simulink model "swim_12B_with_contracts"  (R2019b)
settings: Solver=FixedStepDiscrete  StartTime=0.0  StopTime=10.0  RelTol=1e-3  EnableMultiTasking=on
model workspace (MAT data in the model file):
  ContractValidatorBlocksMap = containers.Map
  ContractValidatorBlocksMap.serialization.keys = {'swim_12B_with_contracts/swim_12B_SWIMSpec/validator'}
  ContractValidatorBlocksMap.serialization.values{1}.block = 'swim_12B_with_contracts/swim_12B_SWIMSpec/validator'
  ContractValidatorBlocksMap.serialization.values{1}.assumePorts = 1
  ContractValidatorBlocksMap.serialization.values{1}.guaranteePorts = 3
  ContractValidatorBlocksMap.serialization.values{1}.modeBlocksPorts = 0
  ContractValidatorBlocksMap.serialization.values{1}.portHandles.Inport = [713.000976562 714.000976562 715.000976562 716.000976562]
  ContractValidatorBlocksMap.serialization.values{1}.portHandles.Outport = 717.000976562
  ContractValidatorBlocksMap.serialization.values{1}.portHandles.Enable = []
  ContractValidatorBlocksMap.serialization.values{1}.portHandles.Trigger = []
  ContractValidatorBlocksMap.serialization.values{1}.portHandles.State = []
  ContractValidatorBlocksMap.serialization.values{1}.portHandles.LConn = []
  ContractValidatorBlocksMap.serialization.values{1}.portHandles.RConn = []
  ContractValidatorBlocksMap.serialization.values{1}.portHandles.Ifaction = []
  ContractValidatorBlocksMap.serialization.values{1}.portHandles.Reset = []
  ContractValidatorBlocksMap.serialization.values{1}.portConnectivity(1).Type = '1'
  ContractValidatorBlocksMap.serialization.values{1}.portConnectivity(1).Position = [1210 730]
  ContractValidatorBlocksMap.serialization.values{1}.portConnectivity(1).SrcBlock = 336.034667969
  ContractValidatorBlocksMap.serialization.values{1}.portConnectivity(1).SrcPort = 0
  ContractValidatorBlocksMap.serialization.values{1}.portConnectivity(1).DstBlock = []
  ContractValidatorBlocksMap.serialization.values{1}.portConnectivity(1).DstPort = []
  ContractValidatorBlocksMap.serialization.values{1}.portConnectivity(2).Type = '2'
  ContractValidatorBlocksMap.serialization.values{1}.portConnectivity(2).Position = [1210 775]
  ContractValidatorBlocksMap.serialization.values{1}.portConnectivity(2).SrcBlock = 340.034667969
  ContractValidatorBlocksMap.serialization.values{1}.portConnectivity(2).SrcPort = 0
  ContractValidatorBlocksMap.serialization.values{1}.portConnectivity(2).DstBlock = []
  ContractValidatorBlocksMap.serialization.values{1}.portConnectivity(2).DstPort = []
  ContractValidatorBlocksMap.serialization.values{1}.portConnectivity(3).Type = '3'
  ContractValidatorBlocksMap.serialization.values{1}.portConnectivity(3).Position = [1210 820]
  ContractValidatorBlocksMap.serialization.values{1}.portConnectivity(3).SrcBlock = 344.034667969
  ContractValidatorBlocksMap.serialization.values{1}.portConnectivity(3).SrcPort = 0
  ContractValidatorBlocksMap.serialization.values{1}.portConnectivity(3).DstBlock = []
  ContractValidatorBlocksMap.serialization.values{1}.portConnectivity(3).DstPort = []
  ContractValidatorBlocksMap.serialization.values{1}.portConnectivity(4).Type = '4'
  ContractValidatorBlocksMap.serialization.values{1}.portConnectivity(4).Position = [1210 865]
  ContractValidatorBlocksMap.serialization.values{1}.portConnectivity(4).SrcBlock = 348.034667969
  ContractValidatorBlocksMap.serialization.values{1}.portConnectivity(4).SrcPort = 0
  ContractValidatorBlocksMap.serialization.values{1}.portConnectivity(4).DstBlock = []
  ContractValidatorBlocksMap.serialization.values{1}.portConnectivity(4).DstPort = []
  ContractValidatorBlocksMap.serialization.values{1}.portConnectivity(5).Type = '1'
  ContractValidatorBlocksMap.serialization.values{1}.portConnectivity(5).Position = [1250 800]
  ContractValidatorBlocksMap.serialization.values{1}.portConnectivity(5).SrcBlock = []
  ContractValidatorBlocksMap.serialization.values{1}.portConnectivity(5).SrcPort = []
  ContractValidatorBlocksMap.serialization.values{1}.portConnectivity(5).DstBlock = 379.034667969
  ContractValidatorBlocksMap.serialization.values{1}.portConnectivity(5).DstPort = 0
  ContractValidatorBlocksMap.serialization.uniformity = 0
  ContractValidatorBlocksMap.serialization.keyType = 'char'
  ContractValidatorBlocksMap.serialization.valueType = 'any'
undefined symbols (not defined in the file): contractAfterSimulation, ContractAssumeBlock, contractBeforeSimulation, ContractBlock, ContractGuaranteeBlock, ContractValidatorBlock, E_DI_CATI, E_DI_DOWN_OR_LOCKED, E_DI_UP_AND_NORMAL, E_MUX_ENABLED, E_OLC_INTERLOCK_NOT_FAILED, E_SWIM_ALLOWED, E_SWIM_NOT_ALLOWED, E_SWIM_WARNING_OFF, E_SWIM_WARNING_ON, saveValidatorParameters
libraries: cocosimLibs x3
settings Model: Creator=belottr  LastModifiedBy=hbourbou
settings DataIOCC: LimitDataPoints=on  SaveFormat=Array  ReturnWorkspaceOutputs=off
settings OptimizationCC: DefaultParameterBehavior=Inlined  ExpressionDepthLimit=2147483647  LifeSpan=inf
settings DebuggingCC: UnderspecifiedInitializationDetection=Classic  MergeDetectMultiDrivingBlocksExec=none  SolverPrmCheckMsg=warning  StateNameClashWarn=warning  SFUnexpectedBacktrackingDiag=warning  SFNoUnconditionalDefaultTransitionDiag=warning  SFExecutionAtInitializationDiag=none  ArithmeticOperatorsInVariantConditions=warning
settings HardwareCC: ProdBitPerPointer=32  ProdBitPerSizeT=32  ProdBitPerPtrDiffT=32  ProdLargestAtomicFloat=None  ProdIntDivRoundTo=Undefined  ProdEndianess=Unspecified  ProdWordSize=32  ProdHWDeviceType=32-bit Generic
settings ModelReferenceCC: UpdateModelReferenceTargets=IfOutOfDate  PropagateSignalLabelsOutOfModel=off
settings SFSimCC: SimUseLocalCustomCode=off  CustomCodeUndefinedFunction=UseInterfaceOnly
settings RTWCC: RTWUseLocalCustomCode=off
settings CodeAppCC: StateflowObjectComments=on
settings GRTTargetCC: TargetLangStandard=C89/C90 (ANSI)  GeneratePreprocessorConditionals=Disable all
settings ConfigComp: CovMetricSettings=dw  CovHtmlReporting=on  CovSaveCumulativeToWorkspaceVar=on  CovSaveSingleToWorkspaceVar=on  CovExternalEMLEnable=off

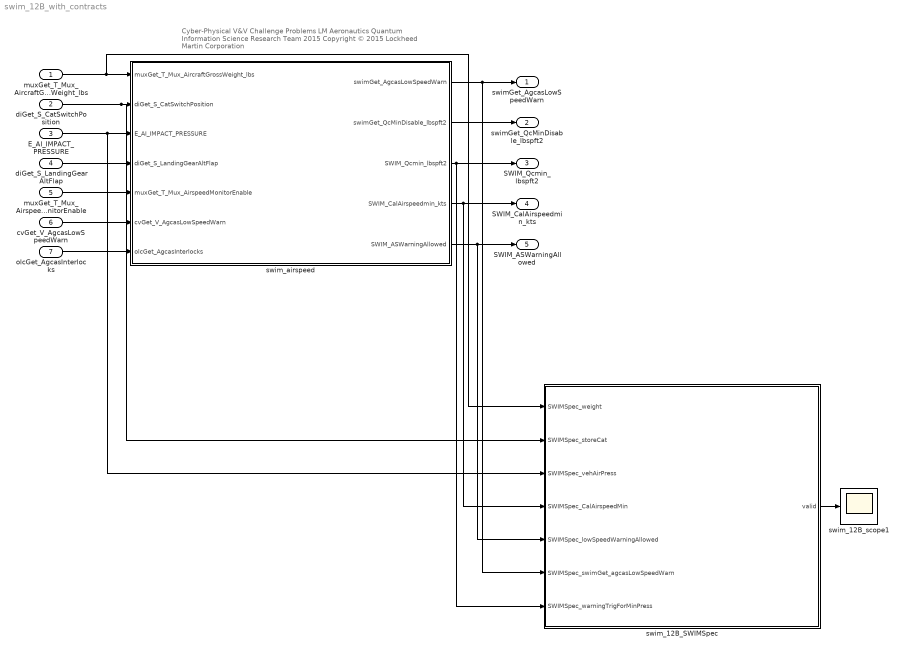
== system swim_12B_with_contracts ==
  note: Cyber-Physical V&V Challenge Problems
      | LM Aeronautics Quantum Information Science Research Team 2015
      | Copyright © 2015 Lockheed Martin Corporation
  muxGet_T_Mux_AircraftGrossWeight_lbs : Inport  OutDataTypeStr=double
  diGet_S_CatSwitchPosition : Inport  Port=2  OutDataTypeStr=int32
  E_AI_IMPACT_PRESSURE : Inport  Port=3  OutDataTypeStr=double
  diGet_S_LandingGearAltFlap : Inport  Port=4  OutDataTypeStr=boolean
  muxGet_T_Mux_AirspeedMonitorEnable : Inport  Port=5  OutDataTypeStr=boolean
  cvGet_V_AgcasLowSpeedWarn : Inport  Port=6  OutDataTypeStr=boolean
  olcGet_AgcasInterlocks : Inport  Port=7  OutDataTypeStr=boolean
  swim_12B_SWIMSpec : Subsystem  mask(ContractBlock){ContractBlockType=ContractBlock}
      mask init:
      | set_param(gcb, 'LinkStatus', 'none');
      mask DialogControl DescTextVar Prompt: Contract block
      mask Display:
      | text(0.5, 0.5, '{\bf\fontsize{20}Contract}', 'hor', 'center', 'texmode','on');
      | blocks = find_system(gcb, 'LookUnderMasks','all', 'SearchDepth',1,'BlockType','Inport');
      | for i = 1 : length(blocks)
      |     blockName = get_param(blocks(i), 'Name');
      |     [path, blockName] = fileparts(char(blockName));
      |     port_label('input', i, blockName);
      | end
      | 
      | blocks = find_system(gcb, 'LookUnderMasks','all', 'SearchDepth',1,'BlockType','Outport');
      | for i = 1 : length(blocks)
      |     blockName = get_param(blocks(i), 'Name');
      |     [path, blockName] = fileparts(char(blockName));
      |     port_label('output', i, blockName);
      | end
  swim_12B_scope1 : Scope
  swim_airspeed : Subsystem
  swimGet_AgcasLowSpeedWarn : Outport  VectorParamsAs1DForOutWhenUnconnected=off
  swimGet_QcMinDisable_lbspft2 : Outport  Port=2  VectorParamsAs1DForOutWhenUnconnected=off
  SWIM_Qcmin_lbspft2 : Outport  Port=3  VectorParamsAs1DForOutWhenUnconnected=off
  SWIM_CalAirspeedmin_kts : Outport  Port=4  VectorParamsAs1DForOutWhenUnconnected=off
  SWIM_ASWarningAllowed : Outport  Port=5  VectorParamsAs1DForOutWhenUnconnected=off
  wires:
  muxGet_T_Mux_AircraftGrossWeight_lbs/1 -> swim_airspeed/1(muxGet_T_Mux_AircraftGrossWeight_lbs), swim_12B_SWIMSpec/1(SWIMSpec_weight)
  diGet_S_CatSwitchPosition/1 -> swim_airspeed/2(diGet_S_CatSwitchPosition), swim_12B_SWIMSpec/2(SWIMSpec_storeCat)
  E_AI_IMPACT_PRESSURE/1 -> swim_airspeed/3(E_AI_IMPACT_PRESSURE), swim_12B_SWIMSpec/3(SWIMSpec_vehAirPress)
  diGet_S_LandingGearAltFlap/1 -> swim_airspeed/4(diGet_S_LandingGearAltFlap)
  muxGet_T_Mux_AirspeedMonitorEnable/1 -> swim_airspeed/5(muxGet_T_Mux_AirspeedMonitorEnable)
  cvGet_V_AgcasLowSpeedWarn/1 -> swim_airspeed/6(cvGet_V_AgcasLowSpeedWarn)
  olcGet_AgcasInterlocks/1 -> swim_airspeed/7(olcGet_AgcasInterlocks)
  swim_airspeed/3(SWIM_Qcmin_lbspft2) -> SWIM_Qcmin_lbspft2/1, swim_12B_SWIMSpec/7(SWIMSpec_warningTrigForMinPress)
  swim_airspeed/2(swimGet_QcMinDisable_lbspft2) -> swimGet_QcMinDisable_lbspft2/1
  swim_airspeed/1(swimGet_AgcasLowSpeedWarn) -> swim_12B_SWIMSpec/6(SWIMSpec_swimGet_agcasLowSpeedWarn), swimGet_AgcasLowSpeedWarn/1
  swim_airspeed/4(SWIM_CalAirspeedmin_kts) -> SWIM_CalAirspeedmin_kts/1, swim_12B_SWIMSpec/4(SWIMSpec_CalAirspeedMin)
  swim_airspeed/5(SWIM_ASWarningAllowed) -> SWIM_ASWarningAllowed/1, swim_12B_SWIMSpec/5(SWIMSpec_lowSpeedWarningAllowed)
  swim_12B_SWIMSpec/1(valid) -> swim_12B_scope1/1

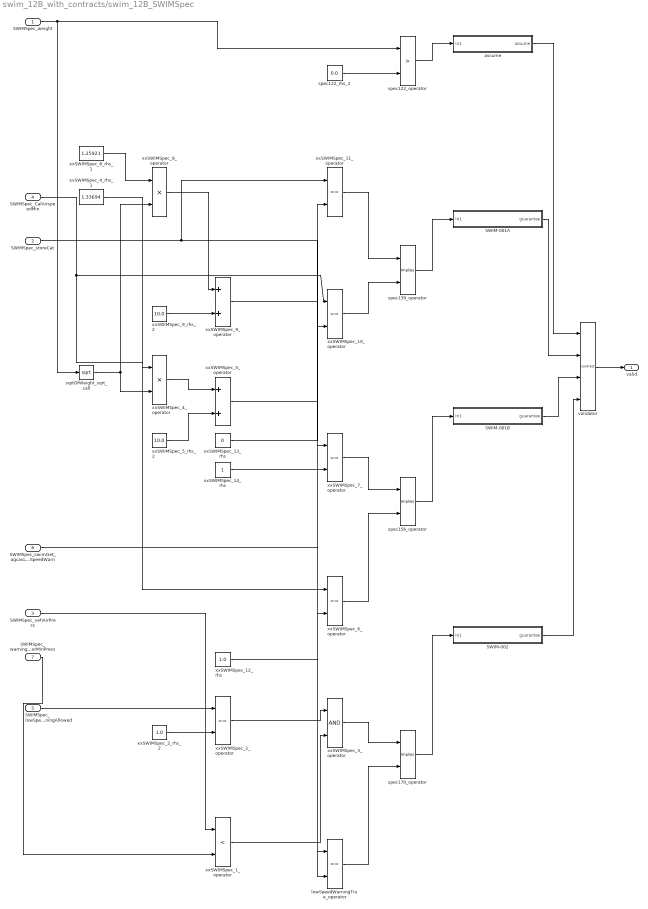
== system swim_12B_with_contracts/swim_12B_SWIMSpec ==
  SWIMSpec_weight : Inport  OutDataTypeStr=double
  SWIMSpec_storeCat : Inport  Port=2
  SWIMSpec_vehAirPress : Inport  Port=3  OutDataTypeStr=double
  SWIMSpec_CalAirspeedMin : Inport  Port=4  OutDataTypeStr=double
  SWIMSpec_lowSpeedWarningAllowed : Inport  Port=5  OutDataTypeStr=double
  SWIMSpec_swimGet_agcasLowSpeedWarn : Inport  Port=6  OutDataTypeStr=double
  SWIMSpec_warningTrigForMinPress : Inport  Port=7  OutDataTypeStr=double
  SWIM-001A : Subsystem  mask(ContractGuaranteeBlock){ContractBlockType=ContractGuaranteeBlock}
      mask init:
      | set_param(gcb, 'LinkStatus', 'none');
      mask DialogControl DescTextVar Prompt: Guarantee block
  SWIM-001B : Subsystem  mask(ContractGuaranteeBlock){ContractBlockType=ContractGuaranteeBlock}
      mask init:
      | set_param(gcb, 'LinkStatus', 'none');
      mask DialogControl DescTextVar Prompt: Guarantee block
  SWIM-002 : Subsystem  mask(ContractGuaranteeBlock){ContractBlockType=ContractGuaranteeBlock}
      mask init:
      | set_param(gcb, 'LinkStatus', 'none');
      mask DialogControl DescTextVar Prompt: Guarantee block
  assume : Subsystem  mask(ContractAssumeBlock){ContractBlockType=ContractAssumeBlock}
      mask init:
      | set_param(gcb, 'LinkStatus', 'none');
      mask DialogControl DescTextVar Prompt: Assume block
  lowSpeedWarningTrue_operator : RelationalOperator  Operator===  OutDataTypeStr=boolean  RndMeth=Simplest
  spec122_operator : RelationalOperator  Operator=>  OutDataTypeStr=boolean  RndMeth=Simplest
  spec122_rhs_2 : Constant  Value=0.0  OutDataTypeStr=double
  spec139_operator : cocosimLibs/Implies  SystemSampleTime=-1  Latency=0  AutoFrameSizeCalculation=off
  spec156_operator : cocosimLibs/Implies  SystemSampleTime=-1  Latency=0  AutoFrameSizeCalculation=off
  spec170_operator : cocosimLibs/Implies  SystemSampleTime=-1  Latency=0  AutoFrameSizeCalculation=off
  sqrtOfWeight_sqrt_call : Sqrt  SaturateOnIntegerOverflow=on
  validator : M-S-Function  LoadFcn=saveValidatorParameters(gcb);  InitFcn=contractBeforeSimulation();  StopFcn=contractAfterSimulation();  FunctionName=contract  mask(ContractValidatorBlock){assumePorts=1, guaranteePorts=3, modePorts=0, ContractBlockType=ContractValidatorBlock, createInportsCheckbox=off}
      mask prompts: assumePorts "Assume ports     :"; guaranteePorts "Guarantee ports :"; modePorts "Mode ports        :"; createInportsCheckbox "Create inports and connect them automatically"
      mask init:
      | set_param(gcb,'LinkStatus','none');
      | contract_callback('inputs_callback',gcb);
      mask DialogControl DescTextVar Prompt: The validator block implements the following logic: <br> <br> <b>Sofar</b>(assume<sub>1</sub> <b>&#8743;</b> assume<sub>2</sub> <b>&#8743;</b> ... assume<sub>k</sub>) <b>&rarr;</b> (guarantee<sub>1</sub> <b>&#8743;</b> guarantee<sub>2</sub> <b>&#8743;</b> ... guarantee<sub>m</sub> <b>&#8743;</b>  mode<sub>1</sub> <b>&#8743;</b> mode<sub>2</sub> <b>&#8743;</b> ... <b>&#8743;</b> mode<sub>n</sub> )<br> where mode<sub>i</sub> = require<sub>i</sub> <b>&rarr;</b> ensure<sub>i</sub>
      mask Display:
      | color('black');
      | port_label('input',1,'assume');
      | port_label('input',2,'guarantee');
      | port_label('input',3,'guarantee');
      | port_label('input',4,'guarantee');
      | port_label('output',1,'valid');
  xxSWIMSpec_10_operator : RelationalOperator  Operator===  OutDataTypeStr=boolean  RndMeth=Simplest
  xxSWIMSpec_11_operator : RelationalOperator  Operator===  OutDataTypeStr=boolean  RndMeth=Simplest
  xxSWIMSpec_12_rhs : Constant  Value=1.0  OutDataTypeStr=double
  xxSWIMSpec_13_rhs : Constant  Value=0  OutDataTypeStr=Inherit: Inherit via back propagation
  xxSWIMSpec_14_rhs : Constant  OutDataTypeStr=Inherit: Inherit via back propagation
  xxSWIMSpec_1_operator : RelationalOperator  Operator=<  OutDataTypeStr=boolean  RndMeth=Simplest
  xxSWIMSpec_2_operator : RelationalOperator  Operator===  OutDataTypeStr=boolean  RndMeth=Simplest
  xxSWIMSpec_2_rhs_2 : Constant  Value=1.0  OutDataTypeStr=double
  xxSWIMSpec_3_operator : Logic  AllPortsSameDT=off  OutDataTypeStr=boolean
  xxSWIMSpec_4_operator : Product  OutDataTypeStr=double
  xxSWIMSpec_4_rhs_1 : Constant  Value=1.33694  OutDataTypeStr=double
  xxSWIMSpec_5_operator : Sum  OutDataTypeStr=double
  xxSWIMSpec_5_rhs_2 : Constant  Value=10.0  OutDataTypeStr=double
  xxSWIMSpec_6_operator : RelationalOperator  Operator===  OutDataTypeStr=boolean  RndMeth=Simplest
  xxSWIMSpec_7_operator : RelationalOperator  Operator===  OutDataTypeStr=boolean  RndMeth=Simplest
  xxSWIMSpec_8_operator : Product  OutDataTypeStr=double
  xxSWIMSpec_8_rhs_1 : Constant  Value=1.25921  OutDataTypeStr=double
  xxSWIMSpec_9_operator : Sum  OutDataTypeStr=double
  xxSWIMSpec_9_rhs_2 : Constant  Value=10.0  OutDataTypeStr=double
  valid : Outport
  wires:
  validator/1 -> valid/1
  xxSWIMSpec_9_rhs_2/1 -> xxSWIMSpec_9_operator/2
  xxSWIMSpec_8_operator/1 -> xxSWIMSpec_9_operator/1
  xxSWIMSpec_8_rhs_1/1 -> xxSWIMSpec_8_operator/1
  xxSWIMSpec_14_rhs/1 -> xxSWIMSpec_7_operator/2
  xxSWIMSpec_5_operator/1 -> xxSWIMSpec_6_operator/2
  xxSWIMSpec_5_rhs_2/1 -> xxSWIMSpec_5_operator/2
  xxSWIMSpec_4_operator/1 -> xxSWIMSpec_5_operator/1
  xxSWIMSpec_4_rhs_1/1 -> xxSWIMSpec_4_operator/1
  xxSWIMSpec_1_operator/1 -> xxSWIMSpec_3_operator/2
  xxSWIMSpec_2_operator/1 -> xxSWIMSpec_3_operator/1
  xxSWIMSpec_2_rhs_2/1 -> xxSWIMSpec_2_operator/2
  SWIMSpec_lowSpeedWarningAllowed/1 -> xxSWIMSpec_2_operator/1
  SWIMSpec_warningTrigForMinPress/1 -> xxSWIMSpec_1_operator/2
  SWIMSpec_vehAirPress/1 -> xxSWIMSpec_1_operator/1
  xxSWIMSpec_13_rhs/1 -> xxSWIMSpec_11_operator/2
  xxSWIMSpec_9_operator/1 -> xxSWIMSpec_10_operator/2
  SWIM-002/1(guarantee) -> validator/4
  SWIM-001B/1(guarantee) -> validator/3
  SWIM-001A/1(guarantee) -> validator/2
  assume/1(assume) -> validator/1
  lowSpeedWarningTrue_operator/1 -> spec170_operator/2
  xxSWIMSpec_3_operator/1 -> spec170_operator/1
  xxSWIMSpec_6_operator/1 -> spec156_operator/2
  xxSWIMSpec_7_operator/1 -> spec156_operator/1
  xxSWIMSpec_10_operator/1 -> spec139_operator/2
  xxSWIMSpec_11_operator/1 -> spec139_operator/1
  spec122_rhs_2/1 -> spec122_operator/2
  xxSWIMSpec_12_rhs/1 -> lowSpeedWarningTrue_operator/2
  SWIMSpec_swimGet_agcasLowSpeedWarn/1 -> lowSpeedWarningTrue_operator/1
  spec170_operator/1 -> SWIM-002/1(In1)
  spec156_operator/1 -> SWIM-001B/1(In1)
  spec139_operator/1 -> SWIM-001A/1(In1)
  spec122_operator/1 -> assume/1(In1)
  SWIMSpec_weight/1 -> sqrtOfWeight_sqrt_call/1, spec122_operator/1
  SWIMSpec_CalAirspeedMin/1 -> xxSWIMSpec_6_operator/1, xxSWIMSpec_10_operator/1
  SWIMSpec_storeCat/1 -> xxSWIMSpec_7_operator/1, xxSWIMSpec_11_operator/1
  sqrtOfWeight_sqrt_call/1 -> xxSWIMSpec_8_operator/2, xxSWIMSpec_4_operator/2

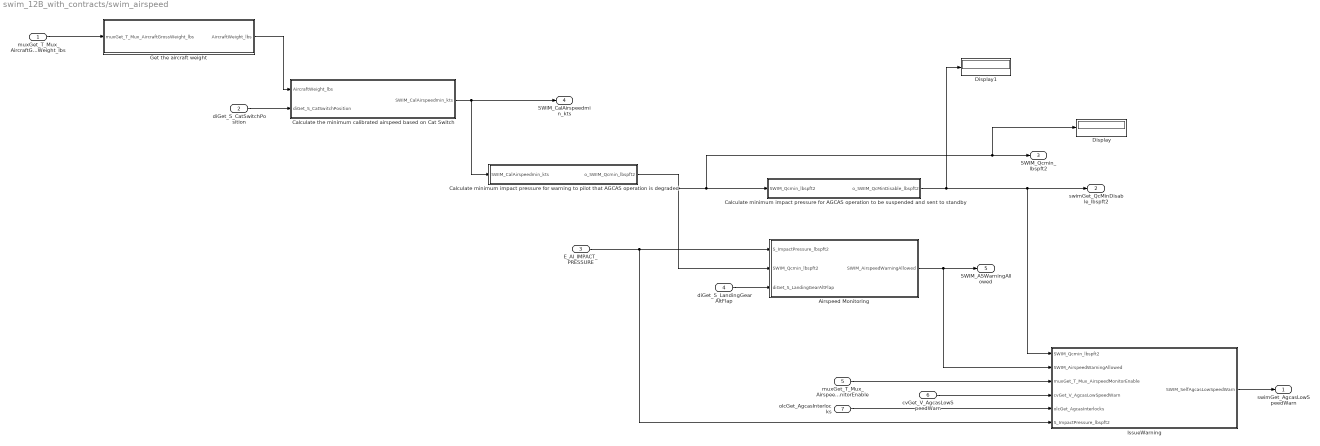
== system swim_12B_with_contracts/swim_airspeed ==
  muxGet_T_Mux_AircraftGrossWeight_lbs : Inport
  diGet_S_CatSwitchPosition : Inport  Port=2
  E_AI_IMPACT_PRESSURE : Inport  Port=3
  diGet_S_LandingGearAltFlap : Inport  Port=4
  muxGet_T_Mux_AirspeedMonitorEnable : Inport  Port=5
  cvGet_V_AgcasLowSpeedWarn : Inport  Port=6
  olcGet_AgcasInterlocks : Inport  Port=7
  Airspeed Monitoring : Subsystem
  Calculate minimum impact pressure for AGCAS operation to be suspended and sent to standby : Subsystem
  Calculate minimum impact pressure for warning to pilot that AGCAS operation is degraded : Subsystem
  Calculate the minimum calibrated airspeed based on Cat Switch : Subsystem
  Display : Display
  Display1 : Display
  Get the aircraft weight : Subsystem
  IssueWarning : Subsystem
  swimGet_AgcasLowSpeedWarn : Outport  VectorParamsAs1DForOutWhenUnconnected=off
  swimGet_QcMinDisable_lbspft2 : Outport  Port=2  VectorParamsAs1DForOutWhenUnconnected=off
  SWIM_Qcmin_lbspft2 : Outport  Port=3  VectorParamsAs1DForOutWhenUnconnected=off
  SWIM_CalAirspeedmin_kts : Outport  Port=4  VectorParamsAs1DForOutWhenUnconnected=off
  SWIM_ASWarningAllowed : Outport  Port=5  VectorParamsAs1DForOutWhenUnconnected=off
  wires:
  muxGet_T_Mux_AircraftGrossWeight_lbs/1 -> Get the aircraft weight/1(muxGet_T_Mux_AircraftGrossWeight_lbs)
  diGet_S_CatSwitchPosition/1 -> Calculate the minimum calibrated airspeed based on Cat Switch/2(diGet_S_CatSwitchPosition)
  Get the aircraft weight/1(AircraftWeight_lbs) -> Calculate the minimum calibrated airspeed based on Cat Switch/1(AircraftWeight_lbs)
  Calculate the minimum calibrated airspeed based on Cat Switch/1(SWIM_CalAirspeedmin_kts) -> Calculate minimum impact pressure for warning to pilot that AGCAS operation is degraded/1(SWIM_CalAirspeedmin_kts), SWIM_CalAirspeedmin_kts/1
  E_AI_IMPACT_PRESSURE/1 -> IssueWarning/6(S_ImpactPressure_lbspft2), Airspeed Monitoring/1(S_ImpactPressure_lbspft2)
  diGet_S_LandingGearAltFlap/1 -> Airspeed Monitoring/3(diGet_S_LandingGearAltFlap)
  IssueWarning/1(SWIM_SelfAgcasLowSpeedWarn) -> swimGet_AgcasLowSpeedWarn/1
  muxGet_T_Mux_AirspeedMonitorEnable/1 -> IssueWarning/3(muxGet_T_Mux_AirspeedMonitorEnable)
  cvGet_V_AgcasLowSpeedWarn/1 -> IssueWarning/4(cvGet_V_AgcasLowSpeedWarn)
  olcGet_AgcasInterlocks/1 -> IssueWarning/5(olcGet_AgcasInterlocks)
  Calculate minimum impact pressure for AGCAS operation to be suspended and sent to standby/1(o_SWIM_QcMinDisable_lbspft2) -> Display1/1, IssueWarning/1(SWIM_Qcmin_lbspft2), swimGet_QcMinDisable_lbspft2/1
  Airspeed Monitoring/1(SWIM_AirspeedWarningAllowed) -> IssueWarning/2(SWIM_AirspeedWarningAllowed), SWIM_ASWarningAllowed/1
  Calculate minimum impact pressure for warning to pilot that AGCAS operation is degraded/1(o_SWIM_Qcmin_lbspft2) -> Airspeed Monitoring/2(SWIM_Qcmin_lbspft2), Display/1, SWIM_Qcmin_lbspft2/1, Calculate minimum impact pressure for AGCAS operation to be suspended and sent to standby/1(SWIM_Qcmin_lbspft2)

== system swim_12B_with_contracts/swim_12B_SWIMSpec/SWIM-001A ==
  In1 : Inport
  guarantee : Outport  OutDataTypeStr=boolean
  wires:
  In1/1 -> guarantee/1

== system swim_12B_with_contracts/swim_12B_SWIMSpec/SWIM-001B ==
  In1 : Inport
  guarantee : Outport  OutDataTypeStr=boolean
  wires:
  In1/1 -> guarantee/1

== system swim_12B_with_contracts/swim_12B_SWIMSpec/SWIM-002 ==
  In1 : Inport
  guarantee : Outport  OutDataTypeStr=boolean
  wires:
  In1/1 -> guarantee/1

== system swim_12B_with_contracts/swim_12B_SWIMSpec/assume ==
  In1 : Inport
  assume : Outport  OutDataTypeStr=boolean
  wires:
  In1/1 -> assume/1

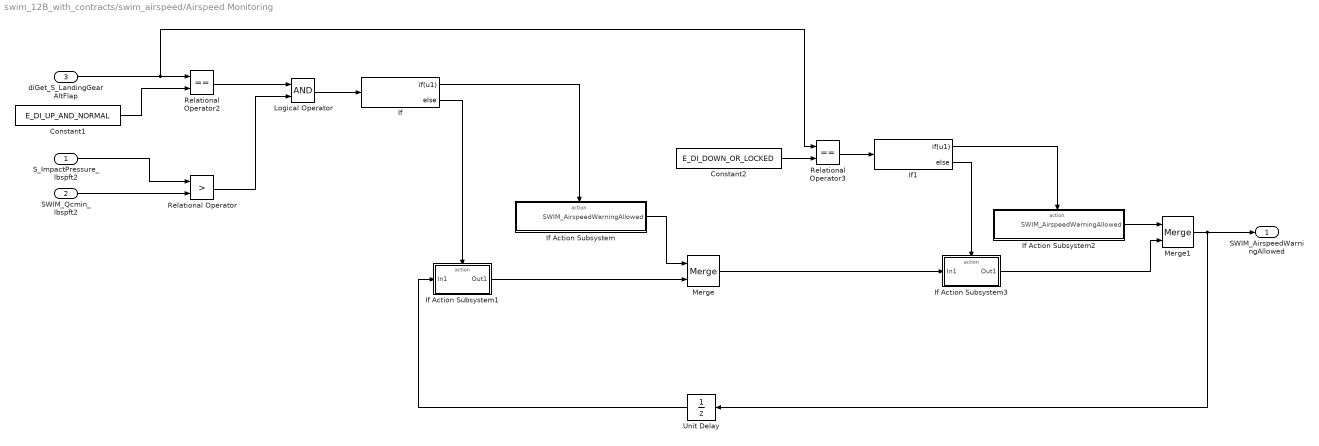
== system swim_12B_with_contracts/swim_airspeed/Airspeed Monitoring ==
  S_ImpactPressure_lbspft2 : Inport
  SWIM_Qcmin_lbspft2 : Inport  Port=2
  diGet_S_LandingGearAltFlap : Inport  Port=3
  Constant1 : Constant  Value=E_DI_UP_AND_NORMAL
  Constant2 : Constant  Value=E_DI_DOWN_OR_LOCKED
  If : If  IfExpression=u1
  If Action Subsystem : Subsystem  TreatAsAtomicUnit=on
  If Action Subsystem1 : Subsystem  TreatAsAtomicUnit=on
  If Action Subsystem2 : Subsystem  TreatAsAtomicUnit=on
  If Action Subsystem3 : Subsystem  TreatAsAtomicUnit=on
  If1 : If  IfExpression=u1
  Logical Operator : Logic  AllPortsSameDT=off  OutDataTypeStr=boolean
  Merge : Merge
  Merge1 : Merge
  Relational Operator : RelationalOperator  Operator=>  OutDataTypeStr=boolean  RndMeth=Nearest
  Relational Operator2 : RelationalOperator  Operator===  OutDataTypeStr=boolean  RndMeth=Nearest
  Relational Operator3 : RelationalOperator  Operator===  OutDataTypeStr=boolean  RndMeth=Nearest
  Unit Delay : UnitDelay  InitialCondition=E_SWIM_NOT_ALLOWED  SampleTime=-1  HasFrameUpgradeWarning=on
  SWIM_AirspeedWarningAllowed : Outport  VectorParamsAs1DForOutWhenUnconnected=off
  wires:
  S_ImpactPressure_lbspft2/1 -> Relational Operator/1
  SWIM_Qcmin_lbspft2/1 -> Relational Operator/2
  diGet_S_LandingGearAltFlap/1 -> Relational Operator3/1, Relational Operator2/1
  Constant1/1 -> Relational Operator2/2
  If/1 -> If Action Subsystem/Action
  If/2 -> If Action Subsystem1/Action
  If Action Subsystem/1(SWIM_AirspeedWarningAllowed) -> Merge/1
  If Action Subsystem1/1(Out1) -> Merge/2
  Constant2/1 -> Relational Operator3/2
  Relational Operator3/1 -> If1/1
  Relational Operator/1 -> Logical Operator/2
  Relational Operator2/1 -> Logical Operator/1
  Logical Operator/1 -> If/1
  If1/1 -> If Action Subsystem2/Action
  If1/2 -> If Action Subsystem3/Action
  If Action Subsystem2/1(SWIM_AirspeedWarningAllowed) -> Merge1/1
  If Action Subsystem3/1(Out1) -> Merge1/2
  Merge/1 -> If Action Subsystem3/1(In1)
  Merge1/1 -> Unit Delay/1, SWIM_AirspeedWarningAllowed/1
  Unit Delay/1 -> If Action Subsystem1/1(In1)

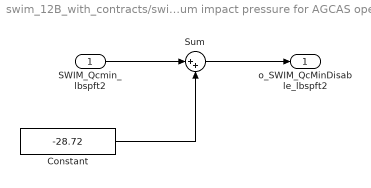
== system swim_12B_with_contracts/swim_airspeed/Calculate minimum impact pressure for AGCAS operation to be suspended and sent to standby ==
  SWIM_Qcmin_lbspft2 : Inport
  Constant : Constant  Value=-28.72
  Sum : Sum  Inputs=|++
  o_SWIM_QcMinDisable_lbspft2 : Outport  VectorParamsAs1DForOutWhenUnconnected=off
  wires:
  SWIM_Qcmin_lbspft2/1 -> Sum/1
  Constant/1 -> Sum/2
  Sum/1 -> o_SWIM_QcMinDisable_lbspft2/1

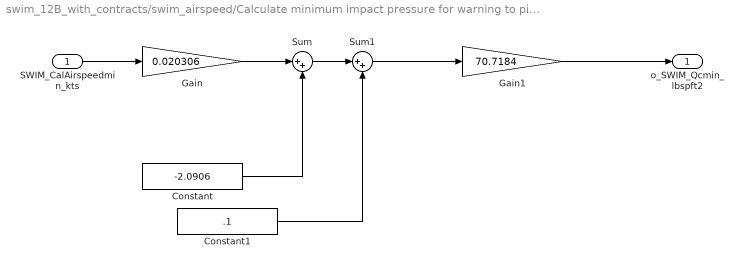
== system swim_12B_with_contracts/swim_airspeed/Calculate minimum impact pressure for warning to pilot that AGCAS operation is degraded ==
  SWIM_CalAirspeedmin_kts : Inport
  Constant : Constant  Value=-2.0906
  Constant1 : Constant  Value=.1
  Gain : Gain  Gain=0.020306
  Gain1 : Gain  Gain=70.7184
  Sum : Sum  Inputs=|++
  Sum1 : Sum  Inputs=|++
  o_SWIM_Qcmin_lbspft2 : Outport  VectorParamsAs1DForOutWhenUnconnected=off
  wires:
  SWIM_CalAirspeedmin_kts/1 -> Gain/1
  Gain/1 -> Sum/1
  Constant/1 -> Sum/2
  Sum/1 -> Sum1/1
  Constant1/1 -> Sum1/2
  Sum1/1 -> Gain1/1
  Gain1/1 -> o_SWIM_Qcmin_lbspft2/1

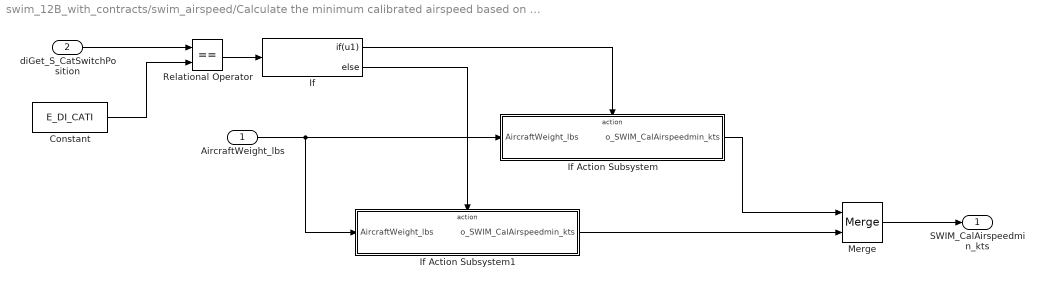
== system swim_12B_with_contracts/swim_airspeed/Calculate the minimum calibrated airspeed based on Cat Switch ==
  AircraftWeight_lbs : Inport
  diGet_S_CatSwitchPosition : Inport  Port=2
  Constant : Constant  Value=E_DI_CATI
  If : If  IfExpression=u1
  If Action Subsystem : Subsystem  TreatAsAtomicUnit=on
  If Action Subsystem1 : Subsystem  TreatAsAtomicUnit=on
  Merge : Merge
  Relational Operator : RelationalOperator  Operator===  OutDataTypeStr=boolean  RndMeth=Nearest
  SWIM_CalAirspeedmin_kts : Outport  VectorParamsAs1DForOutWhenUnconnected=off
  wires:
  If/1 -> If Action Subsystem/Action
  If/2 -> If Action Subsystem1/Action
  If Action Subsystem/1(o_SWIM_CalAirspeedmin_kts) -> Merge/1
  If Action Subsystem1/1(o_SWIM_CalAirspeedmin_kts) -> Merge/2
  Merge/1 -> SWIM_CalAirspeedmin_kts/1
  AircraftWeight_lbs/1 -> If Action Subsystem/1(AircraftWeight_lbs), If Action Subsystem1/1(AircraftWeight_lbs)
  Constant/1 -> Relational Operator/2
  diGet_S_CatSwitchPosition/1 -> Relational Operator/1
  Relational Operator/1 -> If/1

== system swim_12B_with_contracts/swim_airspeed/Get the aircraft weight ==
  muxGet_T_Mux_AircraftGrossWeight_lbs : Inport
  AircraftWeight_lbs : Outport  VectorParamsAs1DForOutWhenUnconnected=off
  wires:
  muxGet_T_Mux_AircraftGrossWeight_lbs/1 -> AircraftWeight_lbs/1

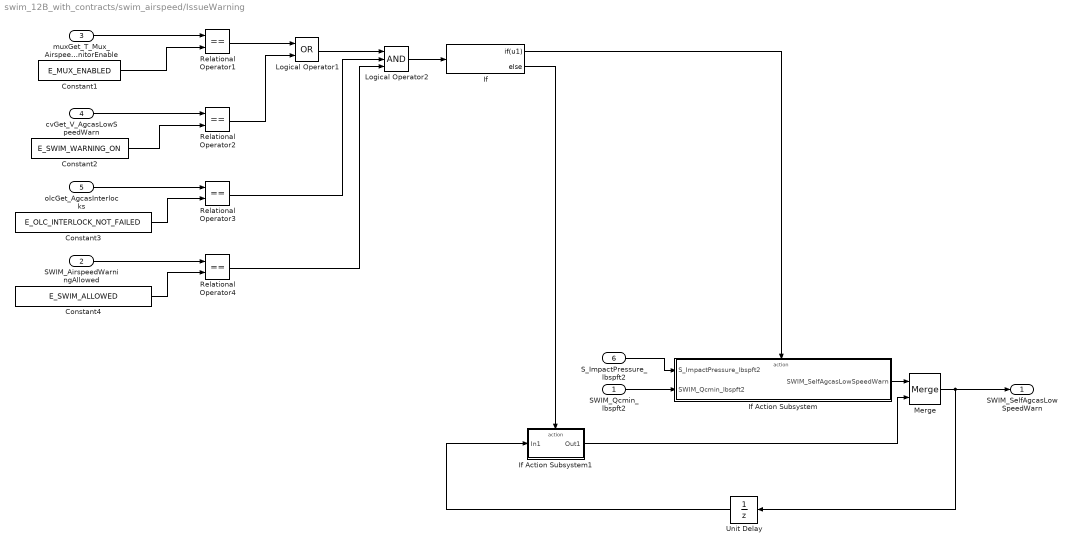
== system swim_12B_with_contracts/swim_airspeed/IssueWarning ==
  SWIM_Qcmin_lbspft2 : Inport
  SWIM_AirspeedWarningAllowed : Inport  Port=2
  muxGet_T_Mux_AirspeedMonitorEnable : Inport  Port=3
  cvGet_V_AgcasLowSpeedWarn : Inport  Port=4
  olcGet_AgcasInterlocks : Inport  Port=5
  S_ImpactPressure_lbspft2 : Inport  Port=6
  Constant1 : Constant  Value=E_MUX_ENABLED
  Constant2 : Constant  Value=E_SWIM_WARNING_ON
  Constant3 : Constant  Value=E_OLC_INTERLOCK_NOT_FAILED
  Constant4 : Constant  Value=E_SWIM_ALLOWED
  If : If  IfExpression=u1
  If Action Subsystem : Subsystem  TreatAsAtomicUnit=on
  If Action Subsystem1 : Subsystem  TreatAsAtomicUnit=on
  Logical Operator1 : Logic  Operator=OR  AllPortsSameDT=off  OutDataTypeStr=boolean
  Logical Operator2 : Logic  Inputs=3  AllPortsSameDT=off  OutDataTypeStr=boolean
  Merge : Merge
  Relational Operator{1..4} (4 alike) : RelationalOperator  Operator===  OutDataTypeStr=boolean  RndMeth=Nearest
  Unit Delay : UnitDelay  InitialCondition=E_SWIM_WARNING_OFF  SampleTime=-1  HasFrameUpgradeWarning=on
  SWIM_SelfAgcasLowSpeedWarn : Outport  VectorParamsAs1DForOutWhenUnconnected=off
  wires:
  muxGet_T_Mux_AirspeedMonitorEnable/1 -> Relational Operator1/1
  cvGet_V_AgcasLowSpeedWarn/1 -> Relational Operator2/1
  Constant2/1 -> Relational Operator2/2
  Constant1/1 -> Relational Operator1/2
  olcGet_AgcasInterlocks/1 -> Relational Operator3/1
  Constant3/1 -> Relational Operator3/2
  SWIM_AirspeedWarningAllowed/1 -> Relational Operator4/1
  Constant4/1 -> Relational Operator4/2
  Relational Operator1/1 -> Logical Operator1/1
  Relational Operator2/1 -> Logical Operator1/2
  Logical Operator1/1 -> Logical Operator2/1
  Relational Operator3/1 -> Logical Operator2/2
  Relational Operator4/1 -> Logical Operator2/3
  Logical Operator2/1 -> If/1
  If/1 -> If Action Subsystem/Action
  If/2 -> If Action Subsystem1/Action
  SWIM_Qcmin_lbspft2/1 -> If Action Subsystem/2(SWIM_Qcmin_lbspft2)
  If Action Subsystem/1(SWIM_SelfAgcasLowSpeedWarn) -> Merge/1
  Merge/1 -> Unit Delay/1, SWIM_SelfAgcasLowSpeedWarn/1
  If Action Subsystem1/1(Out1) -> Merge/2
  Unit Delay/1 -> If Action Subsystem1/1(In1)
  S_ImpactPressure_lbspft2/1 -> If Action Subsystem/1(S_ImpactPressure_lbspft2)

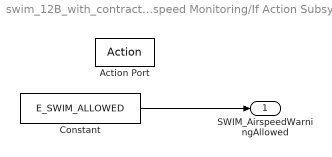
== system swim_12B_with_contracts/swim_airspeed/Airspeed Monitoring/If Action Subsystem ==
  Action Port : ActionPort  ActionPortLabel=if(u1)
  Constant : Constant  Value=E_SWIM_ALLOWED
  SWIM_AirspeedWarningAllowed : Outport  VectorParamsAs1DForOutWhenUnconnected=off
  wires:
  Constant/1 -> SWIM_AirspeedWarningAllowed/1

== system swim_12B_with_contracts/swim_airspeed/Airspeed Monitoring/If Action Subsystem1 ==
  In1 : Inport
  Action Port : ActionPort  ActionPortLabel=else
  Out1 : Outport  VectorParamsAs1DForOutWhenUnconnected=off
  wires:
  In1/1 -> Out1/1

== system swim_12B_with_contracts/swim_airspeed/Airspeed Monitoring/If Action Subsystem2 ==
  Action Port : ActionPort  ActionPortLabel=if(u1)
  Constant : Constant  Value=E_SWIM_NOT_ALLOWED
  SWIM_AirspeedWarningAllowed : Outport  VectorParamsAs1DForOutWhenUnconnected=off
  wires:
  Constant/1 -> SWIM_AirspeedWarningAllowed/1

== system swim_12B_with_contracts/swim_airspeed/Airspeed Monitoring/If Action Subsystem3 ==
  In1 : Inport
  Action Port : ActionPort  ActionPortLabel=else
  Out1 : Outport  VectorParamsAs1DForOutWhenUnconnected=off
  wires:
  In1/1 -> Out1/1

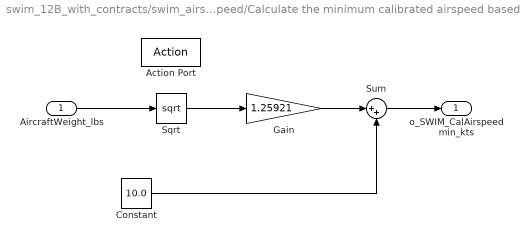
== system swim_12B_with_contracts/swim_airspeed/Calculate the minimum calibrated airspeed based on Cat Switch/If Action Subsystem ==
  AircraftWeight_lbs : Inport
  Action Port : ActionPort  ActionPortLabel=if(u1)
  Constant : Constant  Value=10.0
  Gain : Gain  Gain=1.25921
  Sqrt : Sqrt  SaturateOnIntegerOverflow=on
  Sum : Sum  Inputs=|++
  o_SWIM_CalAirspeedmin_kts : Outport  VectorParamsAs1DForOutWhenUnconnected=off
  wires:
  AircraftWeight_lbs/1 -> Sqrt/1
  Gain/1 -> Sum/1
  Constant/1 -> Sum/2
  Sum/1 -> o_SWIM_CalAirspeedmin_kts/1
  Sqrt/1 -> Gain/1

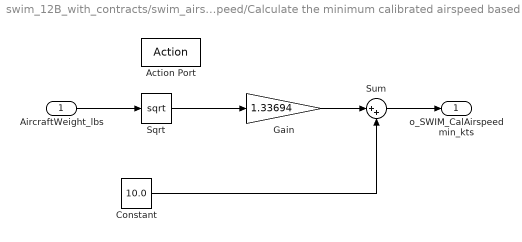
== system swim_12B_with_contracts/swim_airspeed/Calculate the minimum calibrated airspeed based on Cat Switch/If Action Subsystem1 ==
  AircraftWeight_lbs : Inport
  Action Port : ActionPort  ActionPortLabel=else
  Constant : Constant  Value=10.0
  Gain : Gain  Gain=1.33694
  Sqrt : Sqrt  SaturateOnIntegerOverflow=on
  Sum : Sum  Inputs=|++
  o_SWIM_CalAirspeedmin_kts : Outport  VectorParamsAs1DForOutWhenUnconnected=off
  wires:
  Sum/1 -> o_SWIM_CalAirspeedmin_kts/1
  Constant/1 -> Sum/2
  Gain/1 -> Sum/1
  AircraftWeight_lbs/1 -> Sqrt/1
  Sqrt/1 -> Gain/1

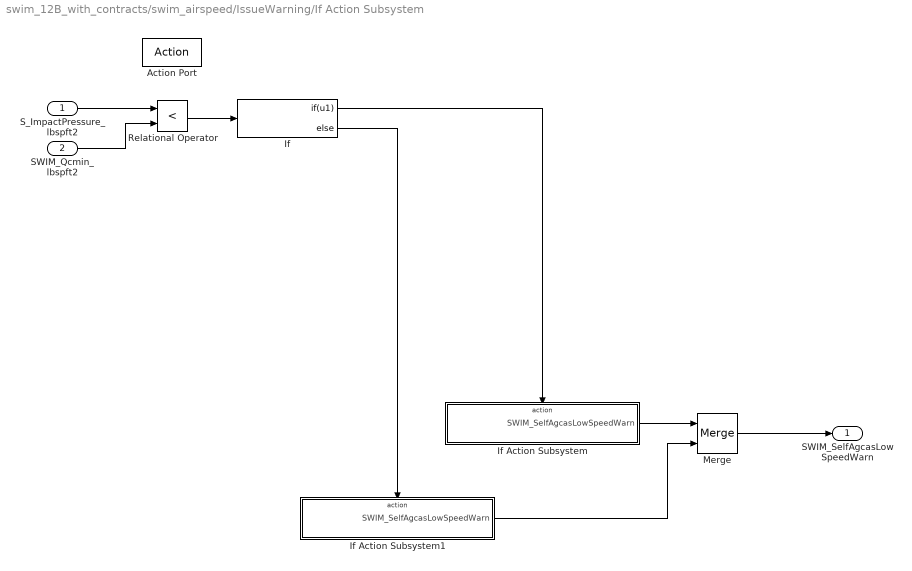
== system swim_12B_with_contracts/swim_airspeed/IssueWarning/If Action Subsystem ==
  S_ImpactPressure_lbspft2 : Inport
  SWIM_Qcmin_lbspft2 : Inport  Port=2
  Action Port : ActionPort  ActionPortLabel=if(u1)
  If : If  IfExpression=u1
  If Action Subsystem : Subsystem  TreatAsAtomicUnit=on
  If Action Subsystem1 : Subsystem  TreatAsAtomicUnit=on
  Merge : Merge
  Relational Operator : RelationalOperator  Operator=<  OutDataTypeStr=boolean  RndMeth=Nearest
  SWIM_SelfAgcasLowSpeedWarn : Outport  VectorParamsAs1DForOutWhenUnconnected=off
  wires:
  S_ImpactPressure_lbspft2/1 -> Relational Operator/1
  SWIM_Qcmin_lbspft2/1 -> Relational Operator/2
  If/1 -> If Action Subsystem/Action
  Relational Operator/1 -> If/1
  Merge/1 -> SWIM_SelfAgcasLowSpeedWarn/1
  If Action Subsystem/1(SWIM_SelfAgcasLowSpeedWarn) -> Merge/1
  If Action Subsystem1/1(SWIM_SelfAgcasLowSpeedWarn) -> Merge/2
  If/2 -> If Action Subsystem1/Action

== system swim_12B_with_contracts/swim_airspeed/IssueWarning/If Action Subsystem1 ==
  In1 : Inport
  Action Port : ActionPort  ActionPortLabel=else
  Out1 : Outport  VectorParamsAs1DForOutWhenUnconnected=off
  wires:
  In1/1 -> Out1/1

== system swim_12B_with_contracts/swim_airspeed/IssueWarning/If Action Subsystem/If Action Subsystem ==
  Action Port : ActionPort  ActionPortLabel=if(u1)
  Constant : Constant  Value=E_SWIM_WARNING_ON
  SWIM_SelfAgcasLowSpeedWarn : Outport  VectorParamsAs1DForOutWhenUnconnected=off
  wires:
  Constant/1 -> SWIM_SelfAgcasLowSpeedWarn/1

== system swim_12B_with_contracts/swim_airspeed/IssueWarning/If Action Subsystem/If Action Subsystem1 ==
  Action Port : ActionPort  ActionPortLabel=else
  Constant : Constant  Value=E_SWIM_WARNING_OFF
  SWIM_SelfAgcasLowSpeedWarn : Outport  VectorParamsAs1DForOutWhenUnconnected=off
  wires:
  Constant/1 -> SWIM_SelfAgcasLowSpeedWarn/1
